simulink model "gm_Model"  (R2025a)
settings: Solver=FixedStepDiscrete  StartTime=0.0  StopTime=80000/fs_in  RelTol=1e-3
undefined symbols (not defined in the file or in its folder): a, b, b_fixp, beta_retanh, c, cos_omega, cos_omega_fixp, diag_count, exp_omega, exp_omega_fixp, fixp_chebacc_frac, fixp_chebacc_ws, fixp_dsp_ws, fixp_eig_frac, fixp_eig_ws, fs_in, group_size, hann_table_fixp, image_seed, image_seed_fixp, J_ROM, k, K_ROM, lap_diags, lap_main, lap_main_fi, lap_offsets, lap_offsets_fi, lap_rest, lap_rest_fi, laplacian_diags_main, laplacian_diags_offsets, laplacian_diags_rest, lut_norm_x, lut_norm_y, magnitude, n_ch, n_layer, n_px, n_px_fi, nf, norm_gain_floor, power_iters, power_norm_scaling_factor_fixp, tau, tau_fixp, theta, theta_fixp
libraries: simulink x59, hdlsllib x36, hdlstreaminglib x4, hdlmdlgenlib x1, matrix_library x1, dspvision x1
(part 5 of 8)

== system gm_Model/DUT_Test/CrossCor/streaming_partition_streamed1/MMul_dot_product_out_bypass ==
  in0 : Inport  OutDataTypeStr=fixdt(1, 18, 13)  PortDimensions=[48]  SampleTime=3.125e-07
      settings: SignalType=complex
  in1 : Inport  Port=2  OutDataTypeStr=boolean  SampleTime=3.125e-07
  MMul_dot_product_out_enb : Switch  Criteria=u2 ~= 0  Threshold=double(0)  OutDataTypeStr=fixdt(1, 18, 13)  SampleTime=3.125e-07  SaturateOnIntegerOverflow=off  InputSameDT=off
  MMul_dot_product_out_state : Delay  DelayLength=double(1)  InitialCondition=0  SampleTime=3.125e-07
  out0 : Outport  OutDataTypeStr=fixdt(1, 18, 13)  PortDimensions=[48]  SampleTime=3.125e-07
      settings: SignalType=complex
  wires:
  in0/1 -> MMul_dot_product_out_enb/1
  in1/1 -> MMul_dot_product_out_enb/2
  MMul_dot_product_out_state/1 -> MMul_dot_product_out_enb/3
  MMul_dot_product_out_enb/1 -> MMul_dot_product_out_state/1, out0/1

== system gm_Model/DUT_Test/CrossCor/streaming_partition_streamed1/Serializer_Subnetwork ==
  in0 : Inport  OutDataTypeStr=fixdt(1, 18, 13)  PortDimensions=[2304 1]  SampleTime=3.125e-07
      settings: SignalType=complex
  in1 : Inport  Port=2  OutDataTypeStr=fixdt(0, 6, 0)  SampleTime=3.125e-07
  ratechange_splitcomp : Demux  Outputs=48
  splitcomp_multiport : MultiPortSwitch  DataPortOrder=Zero-based contiguous  Inputs=48  DiagnosticForDefault=None  zeroidx=on  OutDataTypeStr=fixdt(1, 18, 13)  SampleTime=3.125e-07  SaturateOnIntegerOverflow=off  InputSameDT=off
  out0 : Outport  OutDataTypeStr=fixdt(1, 18, 13)  PortDimensions=[48]  SampleTime=3.125e-07
      settings: SignalType=complex
  wires:
  ratechange_splitcomp/1 -> splitcomp_multiport/2
  ratechange_splitcomp/2 -> splitcomp_multiport/3
  in0/1 -> ratechange_splitcomp/1
  in1/1 -> splitcomp_multiport/1
  ratechange_splitcomp/3 -> splitcomp_multiport/4
  ratechange_splitcomp/4 -> splitcomp_multiport/5
  ratechange_splitcomp/5 -> splitcomp_multiport/6
  ratechange_splitcomp/6 -> splitcomp_multiport/7
  ratechange_splitcomp/10 -> splitcomp_multiport/11
  ratechange_splitcomp/9 -> splitcomp_multiport/10
  ratechange_splitcomp/8 -> splitcomp_multiport/9
  ratechange_splitcomp/7 -> splitcomp_multiport/8
  ratechange_splitcomp/14 -> splitcomp_multiport/15
  ratechange_splitcomp/13 -> splitcomp_multiport/14
  ratechange_splitcomp/12 -> splitcomp_multiport/13
  ratechange_splitcomp/11 -> splitcomp_multiport/12
  ratechange_splitcomp/18 -> splitcomp_multiport/19
  ratechange_splitcomp/17 -> splitcomp_multiport/18
  ratechange_splitcomp/16 -> splitcomp_multiport/17
  ratechange_splitcomp/15 -> splitcomp_multiport/16
  ratechange_splitcomp/22 -> splitcomp_multiport/23
  ratechange_splitcomp/21 -> splitcomp_multiport/22
  ratechange_splitcomp/20 -> splitcomp_multiport/21
  ratechange_splitcomp/19 -> splitcomp_multiport/20
  ratechange_splitcomp/26 -> splitcomp_multiport/27
  ratechange_splitcomp/25 -> splitcomp_multiport/26
  ratechange_splitcomp/24 -> splitcomp_multiport/25
  ratechange_splitcomp/23 -> splitcomp_multiport/24
  ratechange_splitcomp/30 -> splitcomp_multiport/31
  ratechange_splitcomp/29 -> splitcomp_multiport/30
  ratechange_splitcomp/28 -> splitcomp_multiport/29
  ratechange_splitcomp/27 -> splitcomp_multiport/28
  ratechange_splitcomp/34 -> splitcomp_multiport/35
  ratechange_splitcomp/33 -> splitcomp_multiport/34
  ratechange_splitcomp/32 -> splitcomp_multiport/33
  ratechange_splitcomp/31 -> splitcomp_multiport/32
  ratechange_splitcomp/38 -> splitcomp_multiport/39
  ratechange_splitcomp/37 -> splitcomp_multiport/38
  ratechange_splitcomp/36 -> splitcomp_multiport/37
  ratechange_splitcomp/35 -> splitcomp_multiport/36
  ratechange_splitcomp/42 -> splitcomp_multiport/43
  ratechange_splitcomp/41 -> splitcomp_multiport/42
  ratechange_splitcomp/40 -> splitcomp_multiport/41
  ratechange_splitcomp/39 -> splitcomp_multiport/40
  ratechange_splitcomp/46 -> splitcomp_multiport/47
  ratechange_splitcomp/45 -> splitcomp_multiport/46
  ratechange_splitcomp/44 -> splitcomp_multiport/45
  ratechange_splitcomp/43 -> splitcomp_multiport/44
  ratechange_splitcomp/48 -> splitcomp_multiport/49
  ratechange_splitcomp/47 -> splitcomp_multiport/48
  splitcomp_multiport/1 -> out0/1

== system gm_Model/DUT_Test/CrossCor/streaming_partition_streamed1/Serializer_Subnetwork1 ==
  in0 : Inport  OutDataTypeStr=fixdt(1, 18, 13)  PortDimensions=[2304 1]  SampleTime=3.125e-07
      settings: SignalType=complex
  in1 : Inport  Port=2  OutDataTypeStr=fixdt(0, 6, 0)  SampleTime=3.125e-07
  ratechange_splitcomp : Demux  Outputs=48
  splitcomp_multiport : MultiPortSwitch  DataPortOrder=Zero-based contiguous  Inputs=48  DiagnosticForDefault=None  zeroidx=on  OutDataTypeStr=fixdt(1, 18, 13)  SampleTime=3.125e-07  SaturateOnIntegerOverflow=off  InputSameDT=off
  out0 : Outport  OutDataTypeStr=fixdt(1, 18, 13)  PortDimensions=[48]  SampleTime=3.125e-07
      settings: SignalType=complex
  wires:
  in0/1 -> ratechange_splitcomp/1
  in1/1 -> splitcomp_multiport/1
  ratechange_splitcomp/1 -> splitcomp_multiport/2
  ratechange_splitcomp/2 -> splitcomp_multiport/3
  ratechange_splitcomp/3 -> splitcomp_multiport/4
  ratechange_splitcomp/7 -> splitcomp_multiport/8
  ratechange_splitcomp/4 -> splitcomp_multiport/5
  ratechange_splitcomp/5 -> splitcomp_multiport/6
  ratechange_splitcomp/6 -> splitcomp_multiport/7
  ratechange_splitcomp/11 -> splitcomp_multiport/12
  ratechange_splitcomp/10 -> splitcomp_multiport/11
  ratechange_splitcomp/9 -> splitcomp_multiport/10
  ratechange_splitcomp/8 -> splitcomp_multiport/9
  ratechange_splitcomp/15 -> splitcomp_multiport/16
  ratechange_splitcomp/14 -> splitcomp_multiport/15
  ratechange_splitcomp/13 -> splitcomp_multiport/14
  ratechange_splitcomp/12 -> splitcomp_multiport/13
  ratechange_splitcomp/19 -> splitcomp_multiport/20
  ratechange_splitcomp/18 -> splitcomp_multiport/19
  ratechange_splitcomp/17 -> splitcomp_multiport/18
  ratechange_splitcomp/16 -> splitcomp_multiport/17
  ratechange_splitcomp/23 -> splitcomp_multiport/24
  ratechange_splitcomp/22 -> splitcomp_multiport/23
  ratechange_splitcomp/21 -> splitcomp_multiport/22
  ratechange_splitcomp/20 -> splitcomp_multiport/21
  ratechange_splitcomp/27 -> splitcomp_multiport/28
  ratechange_splitcomp/26 -> splitcomp_multiport/27
  ratechange_splitcomp/25 -> splitcomp_multiport/26
  ratechange_splitcomp/24 -> splitcomp_multiport/25
  ratechange_splitcomp/31 -> splitcomp_multiport/32
  ratechange_splitcomp/30 -> splitcomp_multiport/31
  ratechange_splitcomp/29 -> splitcomp_multiport/30
  ratechange_splitcomp/28 -> splitcomp_multiport/29
  ratechange_splitcomp/35 -> splitcomp_multiport/36
  ratechange_splitcomp/34 -> splitcomp_multiport/35
  ratechange_splitcomp/33 -> splitcomp_multiport/34
  ratechange_splitcomp/32 -> splitcomp_multiport/33
  ratechange_splitcomp/39 -> splitcomp_multiport/40
  ratechange_splitcomp/38 -> splitcomp_multiport/39
  ratechange_splitcomp/37 -> splitcomp_multiport/38
  ratechange_splitcomp/36 -> splitcomp_multiport/37
  ratechange_splitcomp/40 -> splitcomp_multiport/41
  ratechange_splitcomp/41 -> splitcomp_multiport/42
  ratechange_splitcomp/44 -> splitcomp_multiport/45
  ratechange_splitcomp/43 -> splitcomp_multiport/44
  ratechange_splitcomp/42 -> splitcomp_multiport/43
  ratechange_splitcomp/48 -> splitcomp_multiport/49
  ratechange_splitcomp/47 -> splitcomp_multiport/48
  ratechange_splitcomp/46 -> splitcomp_multiport/47
  ratechange_splitcomp/45 -> splitcomp_multiport/46
  splitcomp_multiport/1 -> out0/1

== system gm_Model/DUT_Test/CrossCor/streaming_partition_streamed1/counter ==
  globalSchedule : EnablePort  OutDataTypeStr=boolean
  ctr_0_47 : hdlsllib/Sources/HDL Counter  CountType=Count limited  CountInit=double(0)  CountStep=double(1)  CountMax=double(47)  CountFromType=Initial value  CountFrom=double(0)  CountResetPort=off  CountLoadPort=off  CountEnbPort=off  CountDirPort=off  CountHitOutputPort=off  CountDataType=Unsigned  CountWordLen=6  CountFracLen=0  CountSampTime=3.125e-07
  out0 : Outport  OutDataTypeStr=fixdt(0, 6, 0)  SampleTime=3.125e-07  InitialOutput=0
  wires:
  ctr_0_47/1 -> out0/1

== system gm_Model/DUT_Test/CrossCor/streaming_partition_streamed1/tappedDelay ==
  in0 : Inport  OutDataTypeStr=fixdt(1, 18, 13)  PortDimensions=[48]  SampleTime=3.125e-07
      settings: SignalType=complex
  globalSchedule : EnablePort  OutDataTypeStr=boolean
  StateControl : StateControl  StateControl=Synchronous
  tapped_delay : hdlstreaminglib/TappedDelay_VectorInputs  NumDelays=double(47)  vinit=0  DelayOrder=Oldest  includeCurrent=off
  out0 : Outport  OutDataTypeStr=fixdt(1, 18, 13)  PortDimensions=[2256]  SampleTime=3.125e-07  InitialOutput=0
      settings: SignalType=complex
  wires:
  in0/1 -> tapped_delay/1
  tapped_delay/1 -> out0/1

== system gm_Model/DUT_Test/CrossCor/streaming_partition_streamed2/Serializer_Subnetwork ==
  in0 : Inport  OutDataTypeStr=fixdt(1, 18, 13)  PortDimensions=[2304 1]  SampleTime=3.125e-07
      settings: SignalType=complex
  in1 : Inport  Port=2  OutDataTypeStr=fixdt(0, 6, 0)  SampleTime=3.125e-07
  ratechange_splitcomp : Demux  Outputs=48
  splitcomp_multiport : MultiPortSwitch  DataPortOrder=Zero-based contiguous  Inputs=48  DiagnosticForDefault=None  zeroidx=on  OutDataTypeStr=fixdt(1, 18, 13)  SampleTime=3.125e-07  SaturateOnIntegerOverflow=off  InputSameDT=off
  out0 : Outport  OutDataTypeStr=fixdt(1, 18, 13)  PortDimensions=[48]  SampleTime=3.125e-07
      settings: SignalType=complex
  wires:
  ratechange_splitcomp/1 -> splitcomp_multiport/2
  in0/1 -> ratechange_splitcomp/1
  in1/1 -> splitcomp_multiport/1
  ratechange_splitcomp/2 -> splitcomp_multiport/3
  ratechange_splitcomp/3 -> splitcomp_multiport/4
  ratechange_splitcomp/4 -> splitcomp_multiport/5
  ratechange_splitcomp/5 -> splitcomp_multiport/6
  ratechange_splitcomp/9 -> splitcomp_multiport/10
  ratechange_splitcomp/8 -> splitcomp_multiport/9
  ratechange_splitcomp/7 -> splitcomp_multiport/8
  ratechange_splitcomp/6 -> splitcomp_multiport/7
  ratechange_splitcomp/13 -> splitcomp_multiport/14
  ratechange_splitcomp/12 -> splitcomp_multiport/13
  ratechange_splitcomp/11 -> splitcomp_multiport/12
  ratechange_splitcomp/10 -> splitcomp_multiport/11
  ratechange_splitcomp/17 -> splitcomp_multiport/18
  ratechange_splitcomp/16 -> splitcomp_multiport/17
  ratechange_splitcomp/15 -> splitcomp_multiport/16
  ratechange_splitcomp/14 -> splitcomp_multiport/15
  ratechange_splitcomp/21 -> splitcomp_multiport/22
  ratechange_splitcomp/20 -> splitcomp_multiport/21
  ratechange_splitcomp/19 -> splitcomp_multiport/20
  ratechange_splitcomp/18 -> splitcomp_multiport/19
  ratechange_splitcomp/25 -> splitcomp_multiport/26
  ratechange_splitcomp/24 -> splitcomp_multiport/25
  ratechange_splitcomp/23 -> splitcomp_multiport/24
  ratechange_splitcomp/22 -> splitcomp_multiport/23
  ratechange_splitcomp/29 -> splitcomp_multiport/30
  ratechange_splitcomp/28 -> splitcomp_multiport/29
  ratechange_splitcomp/27 -> splitcomp_multiport/28
  ratechange_splitcomp/26 -> splitcomp_multiport/27
  ratechange_splitcomp/33 -> splitcomp_multiport/34
  ratechange_splitcomp/32 -> splitcomp_multiport/33
  ratechange_splitcomp/31 -> splitcomp_multiport/32
  ratechange_splitcomp/30 -> splitcomp_multiport/31
  ratechange_splitcomp/37 -> splitcomp_multiport/38
  ratechange_splitcomp/36 -> splitcomp_multiport/37
  ratechange_splitcomp/35 -> splitcomp_multiport/36
  ratechange_splitcomp/34 -> splitcomp_multiport/35
  ratechange_splitcomp/41 -> splitcomp_multiport/42
  ratechange_splitcomp/40 -> splitcomp_multiport/41
  ratechange_splitcomp/39 -> splitcomp_multiport/40
  ratechange_splitcomp/38 -> splitcomp_multiport/39
  ratechange_splitcomp/45 -> splitcomp_multiport/46
  ratechange_splitcomp/44 -> splitcomp_multiport/45
  ratechange_splitcomp/43 -> splitcomp_multiport/44
  ratechange_splitcomp/42 -> splitcomp_multiport/43
  ratechange_splitcomp/48 -> splitcomp_multiport/49
  ratechange_splitcomp/47 -> splitcomp_multiport/48
  ratechange_splitcomp/46 -> splitcomp_multiport/47
  splitcomp_multiport/1 -> out0/1

== system gm_Model/DUT_Test/CrossCor/streaming_partition_streamed2/Serializer_Subnetwork1 ==
  in0 : Inport  OutDataTypeStr=fixdt(1, 18, 13)  PortDimensions=[2304 1]  SampleTime=3.125e-07
      settings: SignalType=complex
  in1 : Inport  Port=2  OutDataTypeStr=fixdt(0, 6, 0)  SampleTime=3.125e-07
  ratechange_splitcomp : Demux  Outputs=48
  splitcomp_multiport : MultiPortSwitch  DataPortOrder=Zero-based contiguous  Inputs=48  DiagnosticForDefault=None  zeroidx=on  OutDataTypeStr=fixdt(1, 18, 13)  SampleTime=3.125e-07  SaturateOnIntegerOverflow=off  InputSameDT=off
  out0 : Outport  OutDataTypeStr=fixdt(1, 18, 13)  PortDimensions=[48]  SampleTime=3.125e-07
      settings: SignalType=complex
  wires:
  in0/1 -> ratechange_splitcomp/1
  in1/1 -> splitcomp_multiport/1
  ratechange_splitcomp/1 -> splitcomp_multiport/2
  ratechange_splitcomp/2 -> splitcomp_multiport/3
  ratechange_splitcomp/3 -> splitcomp_multiport/4
  ratechange_splitcomp/4 -> splitcomp_multiport/5
  ratechange_splitcomp/5 -> splitcomp_multiport/6
  ratechange_splitcomp/6 -> splitcomp_multiport/7
  ratechange_splitcomp/10 -> splitcomp_multiport/11
  ratechange_splitcomp/9 -> splitcomp_multiport/10
  ratechange_splitcomp/8 -> splitcomp_multiport/9
  ratechange_splitcomp/7 -> splitcomp_multiport/8
  ratechange_splitcomp/14 -> splitcomp_multiport/15
  ratechange_splitcomp/13 -> splitcomp_multiport/14
  ratechange_splitcomp/12 -> splitcomp_multiport/13
  ratechange_splitcomp/11 -> splitcomp_multiport/12
  ratechange_splitcomp/18 -> splitcomp_multiport/19
  ratechange_splitcomp/17 -> splitcomp_multiport/18
  ratechange_splitcomp/16 -> splitcomp_multiport/17
  ratechange_splitcomp/15 -> splitcomp_multiport/16
  ratechange_splitcomp/22 -> splitcomp_multiport/23
  ratechange_splitcomp/21 -> splitcomp_multiport/22
  ratechange_splitcomp/20 -> splitcomp_multiport/21
  ratechange_splitcomp/19 -> splitcomp_multiport/20
  ratechange_splitcomp/23 -> splitcomp_multiport/24
  ratechange_splitcomp/24 -> splitcomp_multiport/25
  ratechange_splitcomp/26 -> splitcomp_multiport/27
  ratechange_splitcomp/25 -> splitcomp_multiport/26
  ratechange_splitcomp/30 -> splitcomp_multiport/31
  ratechange_splitcomp/29 -> splitcomp_multiport/30
  ratechange_splitcomp/28 -> splitcomp_multiport/29
  ratechange_splitcomp/27 -> splitcomp_multiport/28
  splitcomp_multiport/1 -> out0/1
  ratechange_splitcomp/34 -> splitcomp_multiport/35
  ratechange_splitcomp/33 -> splitcomp_multiport/34
  ratechange_splitcomp/32 -> splitcomp_multiport/33
  ratechange_splitcomp/31 -> splitcomp_multiport/32
  ratechange_splitcomp/38 -> splitcomp_multiport/39
  ratechange_splitcomp/37 -> splitcomp_multiport/38
  ratechange_splitcomp/36 -> splitcomp_multiport/37
  ratechange_splitcomp/35 -> splitcomp_multiport/36
  ratechange_splitcomp/47 -> splitcomp_multiport/48
  ratechange_splitcomp/46 -> splitcomp_multiport/47
  ratechange_splitcomp/45 -> splitcomp_multiport/46
  ratechange_splitcomp/44 -> splitcomp_multiport/45
  ratechange_splitcomp/39 -> splitcomp_multiport/40
  ratechange_splitcomp/40 -> splitcomp_multiport/41
  ratechange_splitcomp/41 -> splitcomp_multiport/42
  ratechange_splitcomp/43 -> splitcomp_multiport/44
  ratechange_splitcomp/42 -> splitcomp_multiport/43
  ratechange_splitcomp/48 -> splitcomp_multiport/49

== system gm_Model/DUT_Test/CrossCor/streaming_partition_streamed2/c30_Add_out1_bypass ==
  in0 : Inport  OutDataTypeStr=fixdt(1, 18, 13)  PortDimensions=[48]  SampleTime=3.125e-07
      settings: SignalType=complex
  in1 : Inport  Port=2  OutDataTypeStr=boolean  SampleTime=3.125e-07
  c30_Add_out1_enb : Switch  Criteria=u2 ~= 0  Threshold=double(0)  OutDataTypeStr=fixdt(1, 18, 13)  SampleTime=3.125e-07  SaturateOnIntegerOverflow=off  InputSameDT=off
  c30_Add_out1_state : Delay  DelayLength=double(1)  InitialCondition=0  SampleTime=3.125e-07
  out0 : Outport  OutDataTypeStr=fixdt(1, 18, 13)  PortDimensions=[48]  SampleTime=3.125e-07
      settings: SignalType=complex
  wires:
  in0/1 -> c30_Add_out1_enb/1
  in1/1 -> c30_Add_out1_enb/2
  c30_Add_out1_state/1 -> c30_Add_out1_enb/3
  c30_Add_out1_enb/1 -> c30_Add_out1_state/1, out0/1

== system gm_Model/DUT_Test/CrossCor/streaming_partition_streamed2/counter ==
  globalSchedule : EnablePort  OutDataTypeStr=boolean
  ctr_0_47 : hdlsllib/Sources/HDL Counter  CountType=Count limited  CountInit=double(0)  CountStep=double(1)  CountMax=double(47)  CountFromType=Initial value  CountFrom=double(0)  CountResetPort=off  CountLoadPort=off  CountEnbPort=off  CountDirPort=off  CountHitOutputPort=off  CountDataType=Unsigned  CountWordLen=6  CountFracLen=0  CountSampTime=3.125e-07
  out0 : Outport  OutDataTypeStr=fixdt(0, 6, 0)  SampleTime=3.125e-07  InitialOutput=0
  wires:
  ctr_0_47/1 -> out0/1

== system gm_Model/DUT_Test/CrossCor/streaming_partition_streamed2/tappedDelay ==
  in0 : Inport  OutDataTypeStr=fixdt(1, 18, 13)  PortDimensions=[48]  SampleTime=3.125e-07
      settings: SignalType=complex
  globalSchedule : EnablePort  OutDataTypeStr=boolean
  StateControl : StateControl  StateControl=Synchronous
  tapped_delay : hdlstreaminglib/TappedDelay_VectorInputs  NumDelays=double(47)  vinit=0  DelayOrder=Oldest  includeCurrent=off
  out0 : Outport  OutDataTypeStr=fixdt(1, 18, 13)  PortDimensions=[2256]  SampleTime=3.125e-07  InitialOutput=0
      settings: SignalType=complex
  wires:
  tapped_delay/1 -> out0/1
  in0/1 -> tapped_delay/1

== system gm_Model/DUT_Test/CrossCor/streaming_partition_streamed3/Serializer_Subnetwork ==
  in0 : Inport  OutDataTypeStr=fixdt(1, 18, 13)  PortDimensions=[2304 1]  SampleTime=3.125e-07
      settings: SignalType=complex
  in1 : Inport  Port=2  OutDataTypeStr=fixdt(0, 6, 0)  SampleTime=3.125e-07
  ratechange_splitcomp : Demux  Outputs=48
  splitcomp_multiport : MultiPortSwitch  DataPortOrder=Zero-based contiguous  Inputs=48  DiagnosticForDefault=None  zeroidx=on  OutDataTypeStr=fixdt(1, 18, 13)  SampleTime=3.125e-07  SaturateOnIntegerOverflow=off  InputSameDT=off
  out0 : Outport  OutDataTypeStr=fixdt(1, 18, 13)  PortDimensions=[48]  SampleTime=3.125e-07
      settings: SignalType=complex
  wires:
  in0/1 -> ratechange_splitcomp/1
  in1/1 -> splitcomp_multiport/1
  ratechange_splitcomp/1 -> splitcomp_multiport/2
  ratechange_splitcomp/2 -> splitcomp_multiport/3
  ratechange_splitcomp/3 -> splitcomp_multiport/4
  ratechange_splitcomp/4 -> splitcomp_multiport/5
  ratechange_splitcomp/5 -> splitcomp_multiport/6
  ratechange_splitcomp/9 -> splitcomp_multiport/10
  ratechange_splitcomp/8 -> splitcomp_multiport/9
  ratechange_splitcomp/7 -> splitcomp_multiport/8
  ratechange_splitcomp/6 -> splitcomp_multiport/7
  ratechange_splitcomp/13 -> splitcomp_multiport/14
  ratechange_splitcomp/12 -> splitcomp_multiport/13
  ratechange_splitcomp/11 -> splitcomp_multiport/12
  ratechange_splitcomp/10 -> splitcomp_multiport/11
  ratechange_splitcomp/17 -> splitcomp_multiport/18
  ratechange_splitcomp/16 -> splitcomp_multiport/17
  ratechange_splitcomp/15 -> splitcomp_multiport/16
  ratechange_splitcomp/14 -> splitcomp_multiport/15
  ratechange_splitcomp/21 -> splitcomp_multiport/22
  ratechange_splitcomp/20 -> splitcomp_multiport/21
  ratechange_splitcomp/19 -> splitcomp_multiport/20
  ratechange_splitcomp/18 -> splitcomp_multiport/19
  ratechange_splitcomp/25 -> splitcomp_multiport/26
  ratechange_splitcomp/24 -> splitcomp_multiport/25
  ratechange_splitcomp/23 -> splitcomp_multiport/24
  ratechange_splitcomp/22 -> splitcomp_multiport/23
  ratechange_splitcomp/29 -> splitcomp_multiport/30
  ratechange_splitcomp/28 -> splitcomp_multiport/29
  ratechange_splitcomp/27 -> splitcomp_multiport/28
  ratechange_splitcomp/26 -> splitcomp_multiport/27
  ratechange_splitcomp/33 -> splitcomp_multiport/34
  ratechange_splitcomp/32 -> splitcomp_multiport/33
  ratechange_splitcomp/31 -> splitcomp_multiport/32
  ratechange_splitcomp/30 -> splitcomp_multiport/31
  ratechange_splitcomp/37 -> splitcomp_multiport/38
  ratechange_splitcomp/36 -> splitcomp_multiport/37
  ratechange_splitcomp/35 -> splitcomp_multiport/36
  ratechange_splitcomp/34 -> splitcomp_multiport/35
  ratechange_splitcomp/41 -> splitcomp_multiport/42
  ratechange_splitcomp/40 -> splitcomp_multiport/41
  ratechange_splitcomp/39 -> splitcomp_multiport/40
  ratechange_splitcomp/38 -> splitcomp_multiport/39
  ratechange_splitcomp/45 -> splitcomp_multiport/46
  ratechange_splitcomp/44 -> splitcomp_multiport/45
  ratechange_splitcomp/43 -> splitcomp_multiport/44
  ratechange_splitcomp/42 -> splitcomp_multiport/43
  ratechange_splitcomp/48 -> splitcomp_multiport/49
  ratechange_splitcomp/47 -> splitcomp_multiport/48
  ratechange_splitcomp/46 -> splitcomp_multiport/47
  splitcomp_multiport/1 -> out0/1

== system gm_Model/DUT_Test/CrossCor/streaming_partition_streamed3/Serializer_Subnetwork1 ==
  in0 : Inport  OutDataTypeStr=fixdt(1, 18, 13)  PortDimensions=[2304 1]  SampleTime=3.125e-07
      settings: SignalType=complex
  in1 : Inport  Port=2  OutDataTypeStr=fixdt(0, 6, 0)  SampleTime=3.125e-07
  ratechange_splitcomp : Demux  Outputs=48
  splitcomp_multiport : MultiPortSwitch  DataPortOrder=Zero-based contiguous  Inputs=48  DiagnosticForDefault=None  zeroidx=on  OutDataTypeStr=fixdt(1, 18, 13)  SampleTime=3.125e-07  SaturateOnIntegerOverflow=off  InputSameDT=off
  out0 : Outport  OutDataTypeStr=fixdt(1, 18, 13)  PortDimensions=[48]  SampleTime=3.125e-07
      settings: SignalType=complex
  wires:
  in0/1 -> ratechange_splitcomp/1
  in1/1 -> splitcomp_multiport/1
  ratechange_splitcomp/1 -> splitcomp_multiport/2
  ratechange_splitcomp/2 -> splitcomp_multiport/3
  ratechange_splitcomp/3 -> splitcomp_multiport/4
  ratechange_splitcomp/4 -> splitcomp_multiport/5
  ratechange_splitcomp/5 -> splitcomp_multiport/6
  ratechange_splitcomp/6 -> splitcomp_multiport/7
  ratechange_splitcomp/41 -> splitcomp_multiport/42
  ratechange_splitcomp/10 -> splitcomp_multiport/11
  ratechange_splitcomp/9 -> splitcomp_multiport/10
  ratechange_splitcomp/8 -> splitcomp_multiport/9
  ratechange_splitcomp/7 -> splitcomp_multiport/8
  ratechange_splitcomp/14 -> splitcomp_multiport/15
  ratechange_splitcomp/13 -> splitcomp_multiport/14
  ratechange_splitcomp/12 -> splitcomp_multiport/13
  ratechange_splitcomp/11 -> splitcomp_multiport/12
  ratechange_splitcomp/43 -> splitcomp_multiport/44
  ratechange_splitcomp/42 -> splitcomp_multiport/43
  ratechange_splitcomp/18 -> splitcomp_multiport/19
  ratechange_splitcomp/17 -> splitcomp_multiport/18
  ratechange_splitcomp/16 -> splitcomp_multiport/17
  ratechange_splitcomp/15 -> splitcomp_multiport/16
  ratechange_splitcomp/22 -> splitcomp_multiport/23
  ratechange_splitcomp/21 -> splitcomp_multiport/22
  ratechange_splitcomp/20 -> splitcomp_multiport/21
  ratechange_splitcomp/19 -> splitcomp_multiport/20
  ratechange_splitcomp/26 -> splitcomp_multiport/27
  ratechange_splitcomp/25 -> splitcomp_multiport/26
  ratechange_splitcomp/24 -> splitcomp_multiport/25
  ratechange_splitcomp/23 -> splitcomp_multiport/24
  ratechange_splitcomp/30 -> splitcomp_multiport/31
  ratechange_splitcomp/29 -> splitcomp_multiport/30
  ratechange_splitcomp/28 -> splitcomp_multiport/29
  ratechange_splitcomp/27 -> splitcomp_multiport/28
  ratechange_splitcomp/34 -> splitcomp_multiport/35
  ratechange_splitcomp/33 -> splitcomp_multiport/34
  ratechange_splitcomp/32 -> splitcomp_multiport/33
  ratechange_splitcomp/31 -> splitcomp_multiport/32
  ratechange_splitcomp/38 -> splitcomp_multiport/39
  ratechange_splitcomp/37 -> splitcomp_multiport/38
  ratechange_splitcomp/36 -> splitcomp_multiport/37
  ratechange_splitcomp/35 -> splitcomp_multiport/36
  ratechange_splitcomp/39 -> splitcomp_multiport/40
  ratechange_splitcomp/40 -> splitcomp_multiport/41
  ratechange_splitcomp/47 -> splitcomp_multiport/48
  ratechange_splitcomp/46 -> splitcomp_multiport/47
  ratechange_splitcomp/45 -> splitcomp_multiport/46
  ratechange_splitcomp/44 -> splitcomp_multiport/45
  ratechange_splitcomp/48 -> splitcomp_multiport/49
  splitcomp_multiport/1 -> out0/1

== system gm_Model/DUT_Test/CrossCor/streaming_partition_streamed3/c15_DataInSW_out1_bypass ==
  in0 : Inport  OutDataTypeStr=fixdt(1, 18, 13)  PortDimensions=[48]  SampleTime=3.125e-07
      settings: SignalType=complex
  in1 : Inport  Port=2  OutDataTypeStr=boolean  SampleTime=3.125e-07
  c15_DataInSW_out1_enb : Switch  Criteria=u2 ~= 0  Threshold=double(0)  OutDataTypeStr=fixdt(1, 18, 13)  SampleTime=3.125e-07  SaturateOnIntegerOverflow=off  InputSameDT=off
  c15_DataInSW_out1_state : Delay  DelayLength=double(1)  InitialCondition=0  SampleTime=3.125e-07
  out0 : Outport  OutDataTypeStr=fixdt(1, 18, 13)  PortDimensions=[48]  SampleTime=3.125e-07
      settings: SignalType=complex
  wires:
  in0/1 -> c15_DataInSW_out1_enb/1
  in1/1 -> c15_DataInSW_out1_enb/2
  c15_DataInSW_out1_state/1 -> c15_DataInSW_out1_enb/3
  c15_DataInSW_out1_enb/1 -> c15_DataInSW_out1_state/1, out0/1

== system gm_Model/DUT_Test/CrossCor/streaming_partition_streamed3/counter ==
  globalSchedule : EnablePort  OutDataTypeStr=boolean
  ctr_0_47 : hdlsllib/Sources/HDL Counter  CountType=Count limited  CountInit=double(0)  CountStep=double(1)  CountMax=double(47)  CountFromType=Initial value  CountFrom=double(0)  CountResetPort=off  CountLoadPort=off  CountEnbPort=off  CountDirPort=off  CountHitOutputPort=off  CountDataType=Unsigned  CountWordLen=6  CountFracLen=0  CountSampTime=3.125e-07
  out0 : Outport  OutDataTypeStr=fixdt(0, 6, 0)  SampleTime=3.125e-07  InitialOutput=0
  wires:
  ctr_0_47/1 -> out0/1

== system gm_Model/DUT_Test/CrossCor/streaming_partition_streamed3/tappedDelay ==
  in0 : Inport  OutDataTypeStr=fixdt(1, 18, 13)  PortDimensions=[48]  SampleTime=3.125e-07
      settings: SignalType=complex
  globalSchedule : EnablePort  OutDataTypeStr=boolean
  StateControl : StateControl  StateControl=Synchronous
  tapped_delay : hdlstreaminglib/TappedDelay_VectorInputs  NumDelays=double(47)  vinit=0  DelayOrder=Oldest  includeCurrent=off
  out0 : Outport  OutDataTypeStr=fixdt(1, 18, 13)  PortDimensions=[2256]  SampleTime=3.125e-07  InitialOutput=0
      settings: SignalType=complex
  wires:
  in0/1 -> tapped_delay/1
  tapped_delay/1 -> out0/1

== system gm_Model/DUT_Test/Goertzel/EnabledGoertzel/Hann ==
  In1 : Inport
  Hann : Lookup_n-D  NumberOfTableDimensions=1  LookupTableObject=''  BreakpointsSpecification=Even spacing  BreakpointsForDimension1=[1:200]  BreakpointsForDimension1FirstPoint=0  BreakpointsForDimension2FirstPoint=10  BreakpointsForDimension2Spacing=12  IndexSearchMethod=Evenly spaced points  Table=hann_table_fixp  TableDataTypeStr=Inherit: Inherit from 'Table data'  InterpMethod=Flat  InternalRulePriority=Speed  OutDataTypeStr=fixdt(0,fixp_input_ws,fixp_input_ws)  RndMeth=Simplest
  Hann_pd1 : Delay  DelayLength=1
  Out1 : Outport
  wires:
  In1/1 -> Hann/1
  Hann/1 -> Hann_pd1/1
  Hann_pd1/1 -> Out1/1

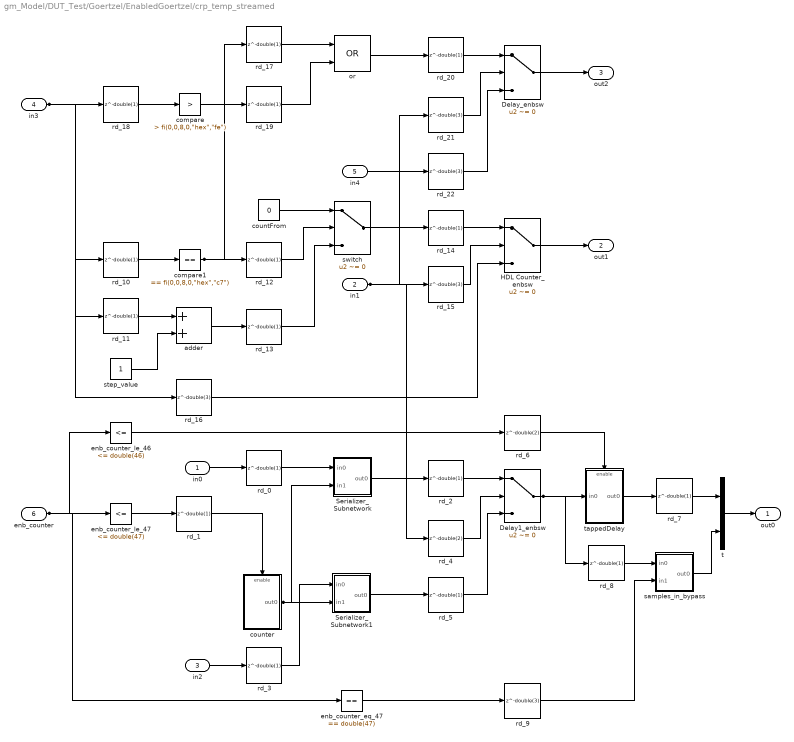
== system gm_Model/DUT_Test/Goertzel/EnabledGoertzel/crp_temp_streamed ==
  in0 : Inport  OutDataTypeStr=fixdt(1, 12, 11)  PortDimensions=[1 48]  SampleTime=3.125e-07
  in1 : Inport  Port=2  OutDataTypeStr=boolean  SampleTime=3.125e-07
  in2 : Inport  Port=3  OutDataTypeStr=fixdt(1, 12, 11)  PortDimensions=[1 48]  SampleTime=3.125e-07
  in3 : Inport  Port=4  OutDataTypeStr=uint8  SampleTime=3.125e-07
  in4 : Inport  Port=5  OutDataTypeStr=boolean  SampleTime=3.125e-07
  enb_counter : Inport  Port=6  OutDataTypeStr=uint8  SampleTime=3.125e-07
  Delay1_enbsw : Switch  Criteria=u2 ~= 0  Threshold=double(0)  OutDataTypeStr=fixdt(1, 12, 11)  SampleTime=3.125e-07  SaturateOnIntegerOverflow=off  InputSameDT=off
  Delay_enbsw : Switch  Criteria=u2 ~= 0  Threshold=double(0)  OutDataTypeStr=boolean  SampleTime=3.125e-07  SaturateOnIntegerOverflow=off  InputSameDT=off
  HDL Counter_enbsw : Switch  Criteria=u2 ~= 0  Threshold=double(0)  OutDataTypeStr=uint8  SampleTime=3.125e-07  SaturateOnIntegerOverflow=off  InputSameDT=off
  Serializer_Subnetwork : Subsystem
  Serializer_Subnetwork1 : Subsystem
  adder : Sum  OutDataTypeStr=uint8  AccumDataTypeStr=uint8  SampleTime=3.125e-07
  compare : simulink/Logic and Bit Operations/Compare To Constant  relop=>  const="fi(0,0,8,0,\"hex\",\"fe\")"  OutDataTypeStr=boolean
  compare1 : simulink/Logic and Bit Operations/Compare To Constant  relop===  const="fi(0,0,8,0,\"hex\",\"c7\")"  OutDataTypeStr=boolean
  countFrom : Constant  Value=0  VectorParams1D=off  OutDataTypeStr=uint8  SampleTime=3.125e-07
  counter : Subsystem
  enb_counter_eq_47 : simulink/Logic and Bit Operations/Compare To Constant  relop===  const=double(47)  OutDataTypeStr=boolean
  enb_counter_le_46 : simulink/Logic and Bit Operations/Compare To Constant  relop=<=  const=double(46)  OutDataTypeStr=boolean
  enb_counter_le_47 : simulink/Logic and Bit Operations/Compare To Constant  relop=<=  const=double(47)  OutDataTypeStr=boolean
  or : Logic  Operator=OR  AllPortsSameDT=off  OutDataTypeStr=boolean  SampleTime=3.125e-07
  rd_{0..3,5,7..8,10..14,17..20} (16 alike) : Delay  DelayLength=double(1)  InitialCondition=0  SampleTime=3.125e-07
  rd_{9,15..16,21..22} (5 alike) : Delay  DelayLength=double(3)  InitialCondition=0  SampleTime=3.125e-07
  rd_4 : Delay  DelayLength=double(2)  InitialCondition=0  SampleTime=3.125e-07
  rd_6 : Delay  DelayLength=double(2)  InitialCondition=0  SampleTime=3.125e-07
  samples_in_bypass : Subsystem
  step_value : Constant  VectorParams1D=off  OutDataTypeStr=uint8  SampleTime=3.125e-07
  switch : Switch  Criteria=u2 ~= 0  Threshold="fi(0,0,1,0,\"hex\",\"0\")"  OutDataTypeStr=uint8  SampleTime=3.125e-07  SaturateOnIntegerOverflow=off  InputSameDT=off
  t : Mux  Inputs=2
  tappedDelay : Subsystem
  out0 : Outport  OutDataTypeStr=fixdt(1, 12, 11)  PortDimensions=[1 48]  SampleTime=3.125e-07
  out1 : Outport  Port=2  OutDataTypeStr=uint8  SampleTime=3.125e-07
  out2 : Outport  Port=3  OutDataTypeStr=boolean  SampleTime=3.125e-07
  wires:
  in3/1 -> rd_16/1, rd_11/1, rd_18/1, rd_10/1
  rd_18/1 -> compare/1
  rd_10/1 -> compare1/1
  enb_counter/1 -> enb_counter_le_47/1, enb_counter_eq_47/1, enb_counter_le_46/1
  rd_11/1 -> adder/1
  rd_13/1 -> switch/3
  adder/1 -> rd_13/1
  step_value/1 -> adder/2
  enb_counter_le_46/1 -> rd_6/1
  enb_counter_le_47/1 -> rd_1/1
  compare/1 -> rd_19/1
  rd_9/1 -> samples_in_bypass/2(in1)
  rd_1/1 -> counter/Enable
  compare1/1 -> rd_17/1, rd_12/1
  rd_16/1 -> HDL Counter_enbsw/3
  in0/1 -> rd_0/1
  in2/1 -> rd_3/1
  Serializer_Subnetwork1/1(out0) -> rd_5/1
  rd_12/1 -> switch/2
  rd_17/1 -> or/1
  rd_20/1 -> Delay_enbsw/1
  rd_19/1 -> or/2
  countFrom/1 -> switch/1
  rd_0/1 -> Serializer_Subnetwork/1(in0)
  counter/1(out0) -> Serializer_Subnetwork1/2(in1), Serializer_Subnetwork/2(in1)
  rd_3/1 -> Serializer_Subnetwork1/1(in0)
  or/1 -> rd_20/1
  in4/1 -> rd_22/1
  switch/1 -> rd_14/1
  in1/1 -> rd_4/1, rd_21/1, rd_15/1
  Serializer_Subnetwork/1(out0) -> rd_2/1
  enb_counter_eq_47/1 -> rd_9/1
  tappedDelay/1(out0) -> rd_7/1
  rd_15/1 -> HDL Counter_enbsw/2
  rd_21/1 -> Delay_enbsw/2
  rd_22/1 -> Delay_enbsw/3
  rd_14/1 -> HDL Counter_enbsw/1
  rd_7/1 -> t/1
  rd_2/1 -> Delay1_enbsw/1
  t/1 -> out0/1
  rd_4/1 -> Delay1_enbsw/2
  rd_5/1 -> Delay1_enbsw/3
  rd_8/1 -> samples_in_bypass/1(in0)
  Delay_enbsw/1 -> out2/1
  HDL Counter_enbsw/1 -> out1/1
  rd_6/1 -> tappedDelay/Enable
  Delay1_enbsw/1 -> rd_8/1, tappedDelay/1(in0)
  samples_in_bypass/1(out0) -> t/2

== system gm_Model/DUT_Test/Goertzel/EnabledGoertzel/crp_temp_streamed1 ==
  in0 : Inport  OutDataTypeStr=boolean  SampleTime=3.125e-07
  in1 : Inport  Port=2  OutDataTypeStr=fixdt(1, 18, 13)  PortDimensions=[1 48]  SampleTime=3.125e-07
  in2 : Inport  Port=3  OutDataTypeStr=boolean  SampleTime=3.125e-07
  in3 : Inport  Port=4  OutDataTypeStr=fixdt(1, 18, 13)  PortDimensions=[1 48]  SampleTime=3.125e-07
  enb_counter : Inport  Port=5  OutDataTypeStr=uint8  SampleTime=3.125e-07
  Constant : Constant  Value=0  OutDataTypeStr=fixdt(1, 18, 13)  SampleTime=3.125e-07
  Delay_enbsw : Switch  Criteria=u2 ~= 0  Threshold=double(0)  OutDataTypeStr=fixdt(1, 18, 13)  SampleTime=3.125e-07  SaturateOnIntegerOverflow=off  InputSameDT=off
  Serializer_Subnetwork : Subsystem
  Serializer_Subnetwork1 : Subsystem
  Switch : Switch  Criteria=u2 ~= 0  Threshold="fi(0,0,1,0,\"hex\",\"0\")"  OutDataTypeStr=fixdt(1, 18, 13)  SampleTime=3.125e-07  SaturateOnIntegerOverflow=off  InputSameDT=off
  Switch_out1_bypass : Subsystem
  counter : Subsystem
  enb_counter_eq_47 : simulink/Logic and Bit Operations/Compare To Constant  relop===  const=double(47)  OutDataTypeStr=boolean
  enb_counter_le_46 : simulink/Logic and Bit Operations/Compare To Constant  relop=<=  const=double(46)  OutDataTypeStr=boolean
  enb_counter_le_47 : simulink/Logic and Bit Operations/Compare To Constant  relop=<=  const=double(47)  OutDataTypeStr=boolean
  rd_{0..1,3..5,9..10} (7 alike) : Delay  DelayLength=double(1)  InitialCondition=0  SampleTime=3.125e-07
  rd_11 : Delay  DelayLength=double(4)  InitialCondition=0  SampleTime=3.125e-07
  rd_2 : Delay  DelayLength=double(2)  InitialCondition=0  SampleTime=3.125e-07
  rd_6 : Delay  DelayLength=double(3)  InitialCondition=0  SampleTime=3.125e-07
  rd_7 : Delay  DelayLength=double(2)  InitialCondition=0  SampleTime=3.125e-07
  rd_8 : Delay  DelayLength=double(3)  InitialCondition=0  SampleTime=3.125e-07
  t : Mux  Inputs=2
  tappedDelay : Subsystem
  out0 : Outport  OutDataTypeStr=fixdt(1, 18, 13)  PortDimensions=[1 48]  SampleTime=3.125e-07
  wires:
  Switch_out1_bypass/1(out0) -> t/2
  rd_0/1 -> Serializer_Subnetwork1/1(in0)
  enb_counter/1 -> enb_counter_eq_47/1, enb_counter_le_47/1, enb_counter_le_46/1
  enb_counter_le_46/1 -> rd_8/1
  in3/1 -> rd_0/1
  enb_counter_le_47/1 -> rd_1/1
  enb_counter_eq_47/1 -> rd_11/1
  rd_8/1 -> tappedDelay/Enable
  rd_1/1 -> counter/Enable
  in2/1 -> rd_2/1
  in1/1 -> rd_5/1
  rd_5/1 -> Serializer_Subnetwork/1(in0)
  rd_7/1 -> Delay_enbsw/3
  counter/1(out0) -> Serializer_Subnetwork/2(in1), Serializer_Subnetwork1/2(in1)
  Serializer_Subnetwork1/1(out0) -> rd_3/1
  Serializer_Subnetwork/1(out0) -> rd_7/1
  Constant/1 -> Switch/1
  rd_2/1 -> Switch/2
  rd_3/1 -> Switch/3
  Switch/1 -> rd_4/1
  in0/1 -> rd_6/1
  rd_10/1 -> Switch_out1_bypass/1(in0)
  rd_11/1 -> Switch_out1_bypass/2(in1)
  rd_9/1 -> t/1
  rd_4/1 -> Delay_enbsw/1
  rd_6/1 -> Delay_enbsw/2
  Delay_enbsw/1 -> rd_10/1, tappedDelay/1(in0)
  tappedDelay/1(out0) -> rd_9/1
  t/1 -> out0/1

== system gm_Model/DUT_Test/Goertzel/EnabledGoertzel/crp_temp_streamed2 ==
  in0 : Inport  OutDataTypeStr=boolean  SampleTime=3.125e-07
  in1 : Inport  Port=2  OutDataTypeStr=fixdt(1, 18, 13)  PortDimensions=[1 48]  SampleTime=3.125e-07
  in2 : Inport  Port=3  OutDataTypeStr=boolean  SampleTime=3.125e-07
  in3 : Inport  Port=4  OutDataTypeStr=fixdt(1, 18, 13)  PortDimensions=[1 48]  SampleTime=3.125e-07
  enb_counter : Inport  Port=5  OutDataTypeStr=uint8  SampleTime=3.125e-07
  Constant : Constant  Value=0  OutDataTypeStr=fixdt(1, 18, 13)  SampleTime=3.125e-07
  Delay_enbsw : Switch  Criteria=u2 ~= 0  Threshold=double(0)  OutDataTypeStr=fixdt(1, 18, 13)  SampleTime=3.125e-07  SaturateOnIntegerOverflow=off  InputSameDT=off
  Serializer_Subnetwork : Subsystem
  Serializer_Subnetwork1 : Subsystem
  Switch : Switch  Criteria=u2 ~= 0  Threshold="fi(0,0,1,0,\"hex\",\"0\")"  OutDataTypeStr=fixdt(1, 18, 13)  SampleTime=3.125e-07  SaturateOnIntegerOverflow=off  InputSameDT=off
  Switch_out1_bypass : Subsystem
  counter : Subsystem
  enb_counter_eq_47 : simulink/Logic and Bit Operations/Compare To Constant  relop===  const=double(47)  OutDataTypeStr=boolean
  enb_counter_le_46 : simulink/Logic and Bit Operations/Compare To Constant  relop=<=  const=double(46)  OutDataTypeStr=boolean
  enb_counter_le_47 : simulink/Logic and Bit Operations/Compare To Constant  relop=<=  const=double(47)  OutDataTypeStr=boolean
  rd_{0..1,3..5,9..10} (7 alike) : Delay  DelayLength=double(1)  InitialCondition=0  SampleTime=3.125e-07
  rd_11 : Delay  DelayLength=double(4)  InitialCondition=0  SampleTime=3.125e-07
  rd_2 : Delay  DelayLength=double(2)  InitialCondition=0  SampleTime=3.125e-07
  rd_6 : Delay  DelayLength=double(3)  InitialCondition=0  SampleTime=3.125e-07
  rd_7 : Delay  DelayLength=double(2)  InitialCondition=0  SampleTime=3.125e-07
  rd_8 : Delay  DelayLength=double(3)  InitialCondition=0  SampleTime=3.125e-07
  t : Mux  Inputs=2
  tappedDelay : Subsystem
  out0 : Outport  OutDataTypeStr=fixdt(1, 18, 13)  PortDimensions=[1 48]  SampleTime=3.125e-07
  wires:
  t/1 -> out0/1
  rd_5/1 -> Serializer_Subnetwork/1(in0)
  rd_1/1 -> counter/Enable
  enb_counter/1 -> enb_counter_le_47/1, enb_counter_eq_47/1, enb_counter_le_46/1
  in0/1 -> rd_6/1
  counter/1(out0) -> Serializer_Subnetwork1/2(in1), Serializer_Subnetwork/2(in1)
  rd_0/1 -> Serializer_Subnetwork1/1(in0)
  enb_counter_le_46/1 -> rd_8/1
  enb_counter_le_47/1 -> rd_1/1
  enb_counter_eq_47/1 -> rd_11/1
  in1/1 -> rd_5/1
  in3/1 -> rd_0/1
  rd_9/1 -> t/1
  in2/1 -> rd_2/1
  Serializer_Subnetwork1/1(out0) -> rd_3/1
  Serializer_Subnetwork/1(out0) -> rd_7/1
  Delay_enbsw/1 -> rd_10/1, tappedDelay/1(in0)
  Constant/1 -> Switch/1
  rd_2/1 -> Switch/2
  rd_3/1 -> Switch/3
  rd_8/1 -> tappedDelay/Enable
  Switch/1 -> rd_4/1
  rd_11/1 -> Switch_out1_bypass/2(in1)
  rd_4/1 -> Delay_enbsw/1
  tappedDelay/1(out0) -> rd_9/1
  rd_6/1 -> Delay_enbsw/2
  rd_10/1 -> Switch_out1_bypass/1(in0)
  rd_7/1 -> Delay_enbsw/3
  Switch_out1_bypass/1(out0) -> t/2

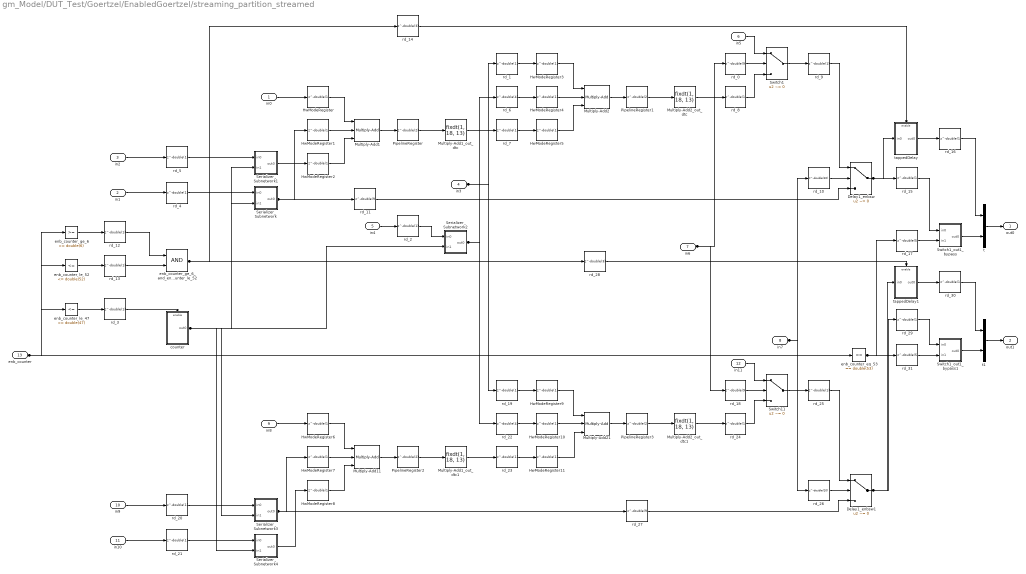
== system gm_Model/DUT_Test/Goertzel/EnabledGoertzel/streaming_partition_streamed ==
  in0 : Inport  OutDataTypeStr=fixdt(1, 18, 13)  SampleTime=3.125e-07
  in1 : Inport  Port=2  OutDataTypeStr=fixdt(1, 18, 13)  PortDimensions=[1 48]  SampleTime=3.125e-07
  in2 : Inport  Port=3  OutDataTypeStr=fixdt(1, 18, 13)  PortDimensions=[1 48]  SampleTime=3.125e-07
  in3 : Inport  Port=4  OutDataTypeStr=fixdt(0, 12, 12)  SampleTime=3.125e-07
  in4 : Inport  Port=5  OutDataTypeStr=fixdt(1, 12, 11)  PortDimensions=[1 48]  SampleTime=3.125e-07
  in5 : Inport  Port=6  OutDataTypeStr=fixdt(1, 18, 13)  SampleTime=3.125e-07
  in6 : Inport  Port=7  OutDataTypeStr=boolean  SampleTime=3.125e-07
  in7 : Inport  Port=8  OutDataTypeStr=boolean  SampleTime=3.125e-07
  in8 : Inport  Port=9  OutDataTypeStr=fixdt(1, 18, 13)  SampleTime=3.125e-07
  in9 : Inport  Port=10  OutDataTypeStr=fixdt(1, 18, 13)  PortDimensions=[1 48]  SampleTime=3.125e-07
  in10 : Inport  Port=11  OutDataTypeStr=fixdt(1, 18, 13)  PortDimensions=[1 48]  SampleTime=3.125e-07
  in11 : Inport  Port=12  OutDataTypeStr=fixdt(1, 18, 13)  SampleTime=3.125e-07
  enb_counter : Inport  Port=13  OutDataTypeStr=uint8  SampleTime=3.125e-07
  Delay1_enbsw : Switch  Criteria=u2 ~= 0  Threshold=double(0)  OutDataTypeStr=fixdt(1, 18, 13)  SampleTime=3.125e-07  SaturateOnIntegerOverflow=off  InputSameDT=off
  Delay1_enbsw1 : Switch  Criteria=u2 ~= 0  Threshold=double(0)  OutDataTypeStr=fixdt(1, 18, 13)  SampleTime=3.125e-07  SaturateOnIntegerOverflow=off  InputSameDT=off
  HwModeRegister{,1..11} (12 alike) : Delay  DelayLength=double(1)  InitialCondition=0  SampleTime=3.125e-07
  Multiply-Add1 : hdlsllib/HDL Operations/Multiply-Add  Function=(a.*b)-c  datatype=fixdt(1, 37, 26)  DoSatur=off  FMA=off
  Multiply-Add11 : hdlsllib/HDL Operations/Multiply-Add  Function=(a.*b)-c  datatype=fixdt(1, 37, 26)  DoSatur=off  FMA=off
  Multiply-Add1_out_dtc : DataTypeConversion  OutDataTypeStr=fixdt(1, 18, 13)  SampleTime=3.125e-07  SaturateOnIntegerOverflow=off  RndMeth=Floor
  Multiply-Add1_out_dtc1 : DataTypeConversion  OutDataTypeStr=fixdt(1, 18, 13)  SampleTime=3.125e-07  SaturateOnIntegerOverflow=off  RndMeth=Floor
  Multiply-Add2 : hdlsllib/HDL Operations/Multiply-Add  Function=c+(a.*b)  datatype=fixdt(1, 29, 23)  DoSatur=off  FMA=off
  Multiply-Add21 : hdlsllib/HDL Operations/Multiply-Add  Function=c+(a.*b)  datatype=fixdt(1, 29, 23)  DoSatur=off  FMA=off
  Multiply-Add2_out_dtc : DataTypeConversion  OutDataTypeStr=fixdt(1, 18, 13)  SampleTime=3.125e-07  SaturateOnIntegerOverflow=off  RndMeth=Floor
  Multiply-Add2_out_dtc1 : DataTypeConversion  OutDataTypeStr=fixdt(1, 18, 13)  SampleTime=3.125e-07  SaturateOnIntegerOverflow=off  RndMeth=Floor
  PipelineRegister{,1..3} (4 alike) : Delay  DelayLength=double(2)  InitialCondition=0  SampleTime=3.125e-07
  Serializer_Subnetwork : Subsystem
  Serializer_Subnetwork1 : Subsystem
  Serializer_Subnetwork2 : Subsystem
  Serializer_Subnetwork3 : Subsystem
  Serializer_Subnetwork4 : Subsystem
  Switch1 : Switch  Criteria=u2 ~= 0  Threshold="fi(0,0,1,0,\"hex\",\"0\")"  OutDataTypeStr=fixdt(1, 18, 13)  SampleTime=3.125e-07  SaturateOnIntegerOverflow=off  InputSameDT=off
  Switch11 : Switch  Criteria=u2 ~= 0  Threshold="fi(0,0,1,0,\"hex\",\"0\")"  OutDataTypeStr=fixdt(1, 18, 13)  SampleTime=3.125e-07  SaturateOnIntegerOverflow=off  InputSameDT=off
  Switch1_out1_bypass : Subsystem
  Switch1_out1_bypass1 : Subsystem
  counter : Subsystem
  enb_counter_eq_53 : simulink/Logic and Bit Operations/Compare To Constant  relop===  const=double(53)  OutDataTypeStr=boolean
  enb_counter_ge_6 : simulink/Logic and Bit Operations/Compare To Constant  relop=>=  const=double(6)  OutDataTypeStr=boolean
  enb_counter_ge_6_and_enb_counter_le_52 : Logic  AllPortsSameDT=off  OutDataTypeStr=boolean  SampleTime=3.125e-07
  enb_counter_le_47 : simulink/Logic and Bit Operations/Compare To Constant  relop=<=  const=double(47)  OutDataTypeStr=boolean
  enb_counter_le_52 : simulink/Logic and Bit Operations/Compare To Constant  relop=<=  const=double(52)  OutDataTypeStr=boolean
  rd_{0,11,18,27} (4 alike) : Delay  DelayLength=double(9)  InitialCondition=0  SampleTime=3.125e-07
  rd_{1..5,7..9,12..13,15..16,19..21,23..25,29..30} (20 alike) : Delay  DelayLength=double(1)  InitialCondition=0  SampleTime=3.125e-07
  rd_10 : Delay  DelayLength=double(10)  InitialCondition=0  SampleTime=3.125e-07
  rd_14 : Delay  DelayLength=double(3)  InitialCondition=0  SampleTime=3.125e-07
  rd_17 : Delay  DelayLength=double(5)  InitialCondition=0  SampleTime=3.125e-07
  rd_22 : Delay  DelayLength=double(4)  InitialCondition=0  SampleTime=3.125e-07
  rd_26 : Delay  DelayLength=double(10)  InitialCondition=0  SampleTime=3.125e-07
  rd_28 : Delay  DelayLength=double(3)  InitialCondition=0  SampleTime=3.125e-07
  rd_31 : Delay  DelayLength=double(5)  InitialCondition=0  SampleTime=3.125e-07
  rd_6 : Delay  DelayLength=double(4)  InitialCondition=0  SampleTime=3.125e-07
  t : Mux  Inputs=2
  t1 : Mux  Inputs=2
  tappedDelay : Subsystem
  tappedDelay1 : Subsystem
  out0 : Outport  OutDataTypeStr=fixdt(1, 18, 13)  PortDimensions=[1 48]  SampleTime=3.125e-07
  out1 : Outport  Port=2  OutDataTypeStr=fixdt(1, 18, 13)  PortDimensions=[1 48]  SampleTime=3.125e-07
  wires:
  in1/1 -> rd_4/1
  enb_counter/1 -> enb_counter_le_52/1, enb_counter_eq_53/1, enb_counter_ge_6/1, enb_counter_le_47/1
  Multiply-Add2/1 -> PipelineRegister1/1
  enb_counter_ge_6/1 -> rd_12/1
  enb_counter_le_47/1 -> rd_3/1
  Serializer_Subnetwork1/1(out0) -> HwModeRegister2/1
  enb_counter_le_52/1 -> rd_13/1
  in3/1 -> rd_19/1, rd_1/1
  in2/1 -> rd_5/1
  rd_12/1 -> enb_counter_ge_6_and_enb_counter_le_52/1
  rd_1/1 -> HwModeRegister3/1
  in0/1 -> HwModeRegister/1
  rd_13/1 -> enb_counter_ge_6_and_enb_counter_le_52/2
  rd_3/1 -> counter/Enable
  HwModeRegister7/1 -> Multiply-Add11/2
  HwModeRegister6/1 -> Multiply-Add11/1
  Serializer_Subnetwork4/1(out0) -> HwModeRegister8/1
  in9/1 -> rd_20/1
  HwModeRegister10/1 -> Multiply-Add21/2
  HwModeRegister9/1 -> Multiply-Add21/1
  in10/1 -> rd_21/1
  rd_4/1 -> Serializer_Subnetwork/1(in0)
  rd_5/1 -> Serializer_Subnetwork1/1(in0)
  enb_counter_ge_6_and_enb_counter_le_52/1 -> rd_14/1, rd_28/1
  rd_11/1 -> Delay1_enbsw/3
  counter/1(out0) -> Serializer_Subnetwork2/2(in1), Serializer_Subnetwork3/2(in1), Serializer_Subnetwork/2(in1), Serializer_Subnetwork1/2(in1), Serializer_Subnetwork4/2(in1)
  rd_20/1 -> Serializer_Subnetwork3/1(in0)
  rd_21/1 -> Serializer_Subnetwork4/1(in0)
  Serializer_Subnetwork/1(out0) -> HwModeRegister1/1, rd_11/1
  in8/1 -> HwModeRegister6/1
  Serializer_Subnetwork3/1(out0) -> HwModeRegister7/1, rd_27/1
  HwModeRegister/1 -> Multiply-Add1/1
  in6/1 -> rd_18/1, rd_0/1
  HwModeRegister1/1 -> Multiply-Add1/2
  Multiply-Add1/1 -> PipelineRegister/1
  HwModeRegister2/1 -> Multiply-Add1/3
  Multiply-Add1_out_dtc/1 -> rd_7/1
  HwModeRegister8/1 -> Multiply-Add11/3
  in4/1 -> rd_2/1
  HwModeRegister5/1 -> Multiply-Add2/3
  Multiply-Add11/1 -> PipelineRegister2/1
  rd_28/1 -> tappedDelay1/Enable
  rd_14/1 -> tappedDelay/Enable
  PipelineRegister/1 -> Multiply-Add1_out_dtc/1
  rd_2/1 -> Serializer_Subnetwork2/1(in0)
  PipelineRegister2/1 -> Multiply-Add1_out_dtc1/1
  PipelineRegister1/1 -> Multiply-Add2_out_dtc/1
  Serializer_Subnetwork2/1(out0) -> rd_22/1, rd_6/1
  HwModeRegister11/1 -> Multiply-Add21/3
  Multiply-Add1_out_dtc1/1 -> rd_23/1
  rd_22/1 -> HwModeRegister10/1
  rd_6/1 -> HwModeRegister4/1
  rd_7/1 -> HwModeRegister5/1
  rd_19/1 -> HwModeRegister9/1
  rd_23/1 -> HwModeRegister11/1
  HwModeRegister4/1 -> Multiply-Add2/2
  HwModeRegister3/1 -> Multiply-Add2/1
  Multiply-Add21/1 -> PipelineRegister3/1
  PipelineRegister3/1 -> Multiply-Add2_out_dtc1/1
  rd_27/1 -> Delay1_enbsw1/3
  Multiply-Add2_out_dtc/1 -> rd_8/1
  Multiply-Add2_out_dtc1/1 -> rd_24/1
  rd_0/1 -> Switch1/2
  in5/1 -> Switch1/1
  rd_8/1 -> Switch1/3
  in11/1 -> Switch11/1
  rd_18/1 -> Switch11/2
  rd_24/1 -> Switch11/3
  Switch1/1 -> rd_9/1
  in7/1 -> rd_26/1, rd_10/1
  Switch11/1 -> rd_25/1
  rd_9/1 -> Delay1_enbsw/1
  rd_10/1 -> Delay1_enbsw/2
  rd_25/1 -> Delay1_enbsw1/1
  rd_26/1 -> Delay1_enbsw1/2
  Delay1_enbsw/1 -> tappedDelay/1(in0), rd_15/1
  enb_counter_eq_53/1 -> rd_31/1, rd_17/1
  Delay1_enbsw1/1 -> rd_29/1, tappedDelay1/1(in0)
  tappedDelay/1(out0) -> rd_16/1
  rd_15/1 -> Switch1_out1_bypass/1(in0)
  rd_17/1 -> Switch1_out1_bypass/2(in1)
  tappedDelay1/1(out0) -> rd_30/1
  rd_29/1 -> Switch1_out1_bypass1/1(in0)
  rd_31/1 -> Switch1_out1_bypass1/2(in1)
  rd_16/1 -> t/1
  Switch1_out1_bypass/1(out0) -> t/2
  rd_30/1 -> t1/1
  Switch1_out1_bypass1/1(out0) -> t1/2
  t/1 -> out0/1
  t1/1 -> out1/1
